simulink subsystem "Regulateur_de_position"  (R2019b)
settings: Solver=VariableStepAuto  StartTime=0.0  StopTime=10.0  RelTol=1e-3
values from neighbouring files (symbols this model uses):
  adc_entrees_resolution = 10    [default_design_data.mat]    (also in dict.sldd = 10.0)
  dac_commande_resolution = 12    [default_design_data.mat]    (also in dict.sldd = 12.0)
  f_echant = 22    [default_design_data.mat]    (also in dict.sldd = 22.0)
  Ki = 0.1408    [default_design_data.mat]    (also in dict.sldd)
  Kp = 0.001    [default_design_data.mat]    (also in dict.sldd)
  V_consigne = 1.8    [default_design_data.mat]    (also in dict.sldd)
libraries: simulink x1
settings Model: Creator=frfoc1  LastModifiedBy=freud

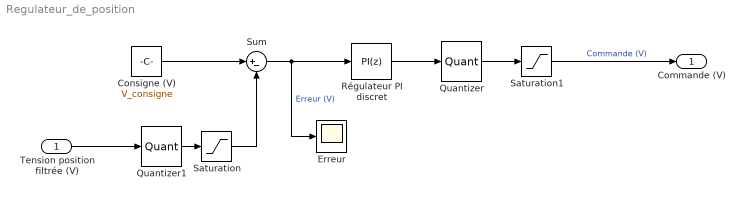
== system Regulateur_de_position ==
  Tension position filtrée (V) : Inport
  Consigne (V) : Constant  Value=V_consigne
  Erreur : Scope
  Quantizer : Quantizer  QuantizationInterval=5/(2^dac_commande_resolution)  LinearizeAsGain=off
  Quantizer1 : Quantizer  QuantizationInterval=5/(2^adc_entrees_resolution)  LinearizeAsGain=off
  Régulateur PI discret : simulink/Continuous/PID Controller  Controller=PI  Form=Parallel  TimeDomain=Discrete-time  SampleTime=1/f_echant  IntegratorMethod=Forward Euler  FilterMethod=Forward Euler  ControllerParametersSource=internal  P=Kp  I=Ki  D=0  UseFilter=on  N=100  TunerSelectOption=Transfer Function Based (PID Tuner App)  InitialConditionSource=internal  InitialConditionForIntegrator=0  InitialConditionForFilter=0  DifferentiatorICPrevScaledInput=0  ExternalReset=none  TrackingMode=off  Kt=1  LimitOutput=on  UpperSaturationLimit=1.6  LowerSaturationLimit=0  LinearizeAsGain=off  AntiWindupMode=clamping  Kb=1  POutMin=[]  POutMax=[]  IOutMin=[]  IOutMax=[]  DOutMin=[]  DOutMax=[]  NOutMin=[]  NOutMax=[]  SumOutMin=[]  SumOutMax=[]  SaturationOutMin=[]  SaturationOutMax=[]  PParamMin=[]  PParamMax=[]  IParamMin=[]  IParamMax=[]  DParamMin=[]  DParamMax=[]  NParamMin=[]  NParamMax=[]  KbParamMin=[]  KbParamMax=[]  KtParamMin=[]  KtParamMax=[]  KbOutMin=[]  KbOutMax=[]  KtOutMin=[]  KtOutMax=[]  IntegratorOutMin=[]  IntegratorOutMax=[]  FilterOutMin=[]  FilterOutMax=[]  SumI1OutMin=[]  SumI1OutMax=[]  SumI2OutMin=[]  SumI2OutMax=[]  SumI3OutMin=[]  SumI3OutMax=[]  SumI4OutMin=[]  SumI4OutMax=[]  SumDOutMin=[]  SumDOutMax=[]  DifferentiatorOutMin=[]  DifferentiatorOutMax=[]  FilterDiffOutCoefMin=[]  FilterDiffOutCoefMax=[]  ReciprocalOutMin=[]  ReciprocalOutMax=[]  SumDenOutMin=[]  SumDenOutMax=[]  SumNumOutMin=[]  SumNumOutMax=[]  DivideOutMin=[]  DivideOutMax=[]  IntegratorContinuousStateAttributes=''  IntegratorStateMustResolveToSignalObject=off  IntegratorRTWStateStorageClass=Auto  FilterContinuousStateAttributes=''  FilterStateMustResolveToSignalObject=off  FilterRTWStateStorageClass=Auto  ParallelPVariant=InternalParameters  IdealPVariant=Disabled  IVariant=InternalParameters  DVariant=Disabled  IntegratorVariant=Discrete  SatVariant=Enabled  AWVariant=DiscClampingParallel  PCopyVariant=Disabled  TRVariant=Disabled  FdbkBlocksVariant=Forward  IdealPFdbkVariant=Disabled  SatFdbkVariant=Disabled  DerivativeFilterVariant=Disabled  NVariant=Disabled  NCopyVariant=Disabled_SignalSpec  FilterICVariant=Disabled  IntegratorICVariant=InternalICs  ExternalResetVariant=Disabled  TRSumVariant=Passthrough  SumFdbkVariant=Disabled  SumVariant=Sum_PI
  Saturation : Saturate  UpperLimit=5  LowerLimit=0
  Saturation1 : Saturate  UpperLimit=1.6  LowerLimit=0
  Sum : Sum  Inputs=|+-
  Commande (V) : Outport
  wires:
  Saturation/1 -> Sum/2
  Quantizer/1 -> Saturation1/1
  Régulateur PI discret/1 -> Quantizer/1
  Quantizer1/1 -> Saturation/1
  Consigne (V)/1 -> Sum/1
  Tension position filtrée (V)/1 -> Quantizer1/1
  Sum/1 -> Erreur/1, Régulateur PI discret/1  "Erreur (V)"
  Saturation1/1 -> Commande (V)/1  "Commande (V)"
